simulink library "BAL_lib"  (Simulink 7.4)
settings: Solver=FixedStepDiscrete  StartTime=0.0  StopTime=Inf  FixedStep=0.01  RelTol=1e-3
undefined symbols (not defined in the file or in its folder): FCM_Charging_St, PACK_Const_CellNumOfPack, SCM_Charging_St
libraries: Defined_Functionality x3
settings Model: Creator=zhaoxiangri  LastModifiedBy=sunsijun

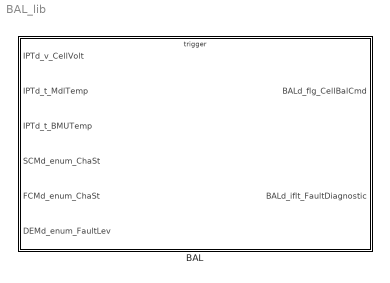
== system BAL_lib ==
  BAL : Subsystem  TreatAsAtomicUnit=on

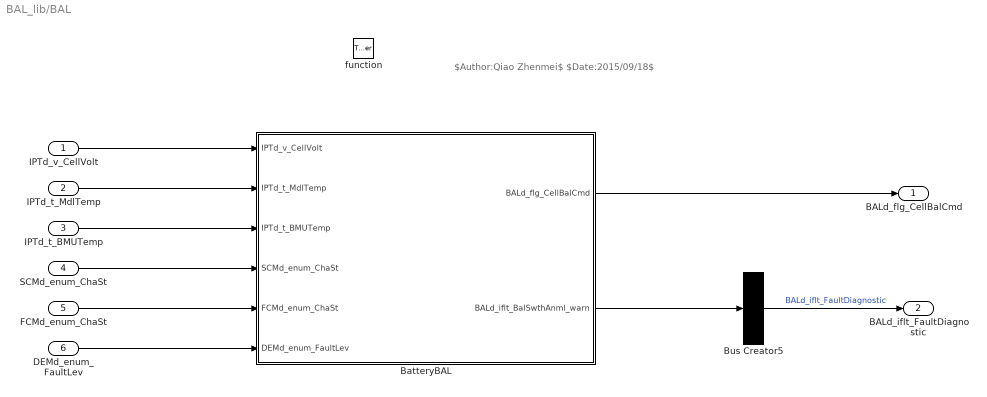
== system BAL_lib/BAL ==
  note: $Author:Qiao Zhenmei$
      | $Date:2015/09/18$
  IPTd_v_CellVolt : Inport  PortDimensions=[1 160]
  IPTd_t_MdlTemp : Inport  Port=2  DataType=single  OutDataTypeStr=single
  IPTd_t_BMUTemp : Inport  Port=3  DataType=single  OutDataTypeStr=single
  SCMd_enum_ChaSt : Inport  Port=4  DataType=uint8  OutDataTypeStr=uint8
  FCMd_enum_ChaSt : Inport  Port=5
  DEMd_enum_FaultLev : Inport  Port=6  DataType=uint8  OutDataTypeStr=uint8
  function : TriggerPort  TriggerType=function-call
  BatteryBAL : Subsystem  TreatAsAtomicUnit=on
  Bus Creator5 : BusCreator  Inputs=1
  BALd_flg_CellBalCmd : Outport
  BALd_iflt_FaultDiagnostic : Outport  Port=2  OutDataType=fixdt(1, 16)  OutScaling=2^0
  wires:
  Bus Creator5/1 -> BALd_iflt_FaultDiagnostic/1  "BALd_iflt_FaultDiagnostic"
  BatteryBAL/2(BALd_iflt_BalSwthAnml_warn) -> Bus Creator5/1
  IPTd_t_BMUTemp/1 -> BatteryBAL/3(IPTd_t_BMUTemp)
  BatteryBAL/1(BALd_flg_CellBalCmd) -> BALd_flg_CellBalCmd/1
  DEMd_enum_FaultLev/1 -> BatteryBAL/6(DEMd_enum_FaultLev)
  IPTd_t_MdlTemp/1 -> BatteryBAL/2(IPTd_t_MdlTemp)
  IPTd_v_CellVolt/1 -> BatteryBAL/1(IPTd_v_CellVolt)
  SCMd_enum_ChaSt/1 -> BatteryBAL/4(SCMd_enum_ChaSt)
  FCMd_enum_ChaSt/1 -> BatteryBAL/5(FCMd_enum_ChaSt)

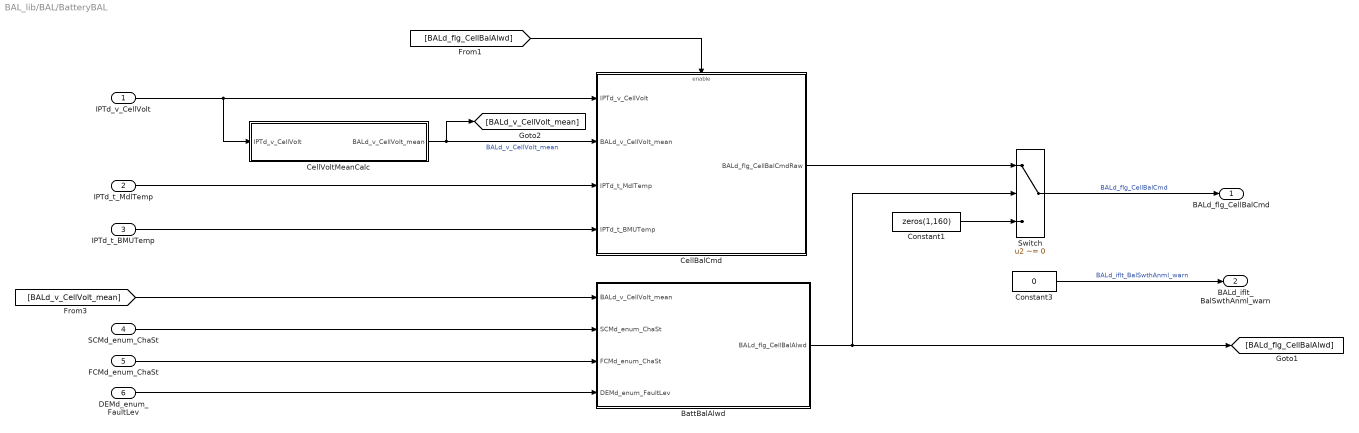
== system BAL_lib/BAL/BatteryBAL ==
  IPTd_v_CellVolt : Inport  DataType=single  OutDataTypeStr=single
  IPTd_t_MdlTemp : Inport  Port=2
  IPTd_t_BMUTemp : Inport  Port=3
  SCMd_enum_ChaSt : Inport  Port=4  DataType=uint8  OutDataTypeStr=uint8
  FCMd_enum_ChaSt : Inport  Port=5
  DEMd_enum_FaultLev : Inport  Port=6
  BattBalAlwd : Subsystem
  CellBalCmd : Subsystem
  CellVoltMeanCalc : Subsystem
  Constant1 : Constant  Value=zeros(1,160)  OutDataTypeMode=boolean  OutDataType=fixdt(1, 16)  OutScaling=2^0  OutDataTypeStr=boolean
  Constant3 : Constant  Value=0  OutDataTypeMode=boolean  OutDataTypeStr=boolean
  Switch : Switch  Criteria=u2 ~= 0  OutDataType=fixdt(1, 16)  OutScaling=2^0
  BALd_flg_CellBalCmd : Outport
  BALd_iflt_BalSwthAnml_warn : Outport  Port=2  OutDataType=fixdt(1, 16)  OutScaling=2^0  InitialOutput=0
  wires:
  [BALd_flg_CellBalAlwd] -> CellBalCmd/Enable
  CellBalCmd/1(BALd_flg_CellBalCmdRaw) -> Switch/1
  Constant1/1 -> Switch/3
  CellVoltMeanCalc/1(BALd_v_CellVolt_mean) -> [BALd_v_CellVolt_mean], CellBalCmd/2(BALd_v_CellVolt_mean)  "BALd_v_CellVolt_mean"
  Constant3/1 -> BALd_iflt_BalSwthAnml_warn/1  "BALd_iflt_BalSwthAnml_warn"
  IPTd_v_CellVolt/1 -> CellVoltMeanCalc/1(IPTd_v_CellVolt), CellBalCmd/1(IPTd_v_CellVolt)
  Switch/1 -> BALd_flg_CellBalCmd/1  "BALd_flg_CellBalCmd"
  IPTd_t_MdlTemp/1 -> CellBalCmd/3(IPTd_t_MdlTemp)
  IPTd_t_BMUTemp/1 -> CellBalCmd/4(IPTd_t_BMUTemp)
  BattBalAlwd/1(BALd_flg_CellBalAlwd) -> [BALd_flg_CellBalAlwd], Switch/2
  [BALd_v_CellVolt_mean] -> BattBalAlwd/1(BALd_v_CellVolt_mean)
  DEMd_enum_FaultLev/1 -> BattBalAlwd/4(DEMd_enum_FaultLev)
  SCMd_enum_ChaSt/1 -> BattBalAlwd/2(SCMd_enum_ChaSt)
  FCMd_enum_ChaSt/1 -> BattBalAlwd/3(FCMd_enum_ChaSt)

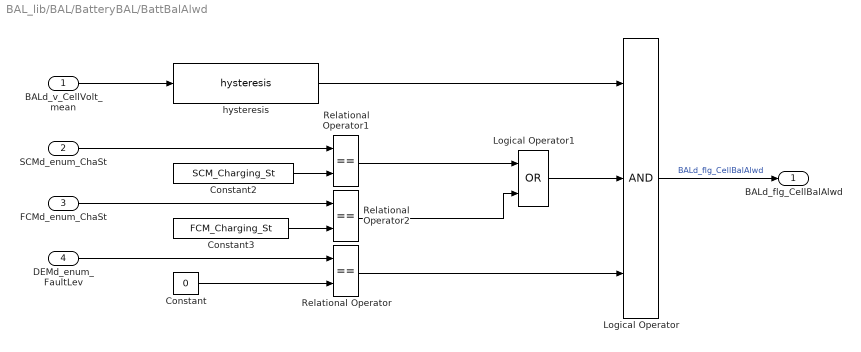
== system BAL_lib/BAL/BatteryBAL/BattBalAlwd ==
  BALd_v_CellVolt_mean : Inport
  SCMd_enum_ChaSt : Inport  Port=2  DataType=uint8  OutDataTypeStr=uint8
  FCMd_enum_ChaSt : Inport  Port=3
  DEMd_enum_FaultLev : Inport  Port=4
  Constant : Constant  Value=0  OutDataTypeMode=uint8  OutDataTypeStr=uint8
  Constant2 : Constant  Value=SCM_Charging_St  OutDataTypeMode=uint8  OutDataTypeStr=uint8
  Constant3 : Constant  Value=FCM_Charging_St  OutDataTypeMode=uint8  OutDataTypeStr=uint8
  Logical Operator : Logic  Inputs=3  AllPortsSameDT=off  OutDataTypeMode=boolean  OutDataTypeStr=boolean
  Logical Operator1 : Logic  Operator=OR  AllPortsSameDT=off  OutDataTypeMode=boolean  LogicDataType=fixdt(0, 8)  OutDataTypeStr=boolean
  Relational Operator : RelationalOperator  Operator===  LogicOutDataTypeMode=boolean  OutDataTypeStr=boolean
  Relational Operator1 : RelationalOperator  Operator===  LogicOutDataTypeMode=boolean  OutDataTypeStr=boolean
  Relational Operator2 : RelationalOperator  Operator===  LogicOutDataTypeMode=boolean  OutDataTypeStr=boolean
  hysteresis : Defined_Functionality/hysteresis  SystemSampleTime=-1  upper_limit=BALc_v_BalCellVoltOn  lower_limit=BALc_v_BalCellVoltOff
      settings: AttributesFormatString=[UPPER_LIMIT=%<upper_limit>]\n[LOWER_LIMIT=%<lower_limit>]
  BALd_flg_CellBalAlwd : Outport
  wires:
  hysteresis/1 -> Logical Operator/1
  Relational Operator2/1 -> Logical Operator1/2
  Logical Operator1/1 -> Logical Operator/2
  Constant3/1 -> Relational Operator2/2
  BALd_v_CellVolt_mean/1 -> hysteresis/1
  Logical Operator/1 -> BALd_flg_CellBalAlwd/1  "BALd_flg_CellBalAlwd"
  Relational Operator/1 -> Logical Operator/3
  Constant/1 -> Relational Operator/2
  DEMd_enum_FaultLev/1 -> Relational Operator/1
  FCMd_enum_ChaSt/1 -> Relational Operator2/1
  Relational Operator1/1 -> Logical Operator1/1
  Constant2/1 -> Relational Operator1/2
  SCMd_enum_ChaSt/1 -> Relational Operator1/1

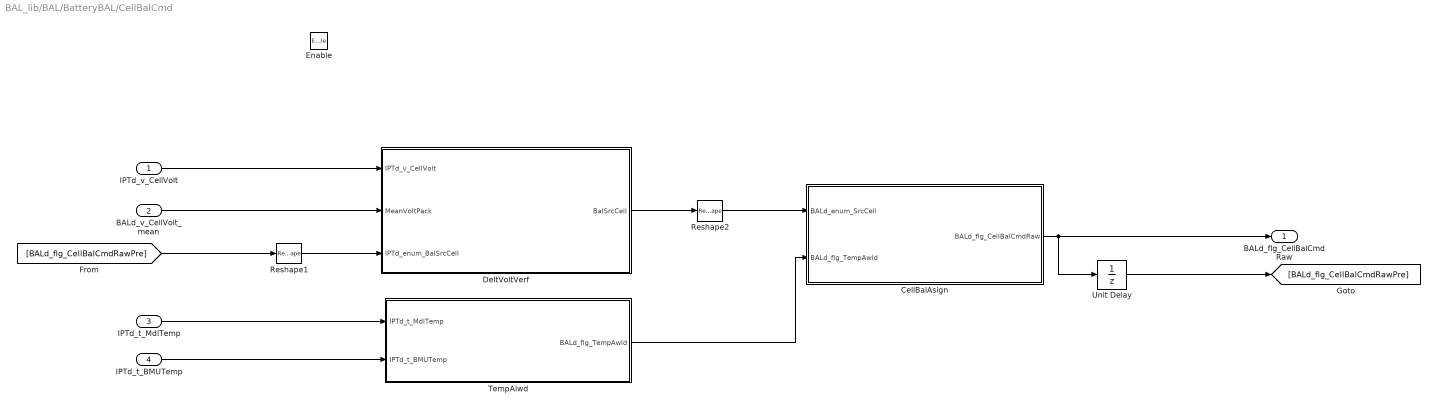
== system BAL_lib/BAL/BatteryBAL/CellBalCmd ==
  IPTd_v_CellVolt : Inport
  BALd_v_CellVolt_mean : Inport  Port=2
  IPTd_t_MdlTemp : Inport  Port=3
  IPTd_t_BMUTemp : Inport  Port=4
  Enable : EnablePort
  CellBalAsign : Subsystem
  DeltVoltVerf : Stateflow chart  TreatAsAtomicUnit=on
  Reshape1 : Reshape  OutputDimensionality=Customize  OutputDimensions=[5,32]
  Reshape2 : Reshape  OutputDimensionality=Row vector (2-D)  OutputDimensions=[40,4]
  TempAlwd : Subsystem
  Unit Delay : UnitDelay  SampleTime=-1
  BALd_flg_CellBalCmdRaw : Outport
  wires:
  [BALd_flg_CellBalCmdRawPre] -> Reshape1/1
  Unit Delay/1 -> [BALd_flg_CellBalCmdRawPre]
  Reshape2/1 -> CellBalAsign/1(BALd_enum_SrcCell)
  Reshape1/1 -> DeltVoltVerf/3(IPTd_enum_BalSrcCell)
  DeltVoltVerf/1(BalSrcCell) -> Reshape2/1
  TempAlwd/1(BALd_flg_TempAwld) -> CellBalAsign/2(BALd_flg_TempAwld)
  IPTd_t_MdlTemp/1 -> TempAlwd/1(IPTd_t_MdlTemp)
  IPTd_t_BMUTemp/1 -> TempAlwd/2(IPTd_t_BMUTemp)
  BALd_v_CellVolt_mean/1 -> DeltVoltVerf/2(MeanVoltPack)
  CellBalAsign/1(BALd_flg_CellBalCmdRaw) -> BALd_flg_CellBalCmdRaw/1, Unit Delay/1
  IPTd_v_CellVolt/1 -> DeltVoltVerf/1(IPTd_v_CellVolt)

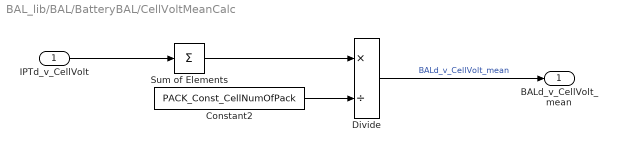
== system BAL_lib/BAL/BatteryBAL/CellVoltMeanCalc ==
  IPTd_v_CellVolt : Inport
  Constant2 : Constant  Value=PACK_Const_CellNumOfPack  OutDataTypeMode=uint8  OutDataTypeStr=uint8
  Divide : Product  Inputs=*/  OutDataType=fixdt(1, 16)  OutScaling=2^-10
  Sum of Elements : Sum  Inputs=+  OutDataType=fixdt(1, 16)  OutScaling=2^-10
  BALd_v_CellVolt_mean : Outport
  wires:
  Divide/1 -> BALd_v_CellVolt_mean/1  "BALd_v_CellVolt_mean"
  IPTd_v_CellVolt/1 -> Sum of Elements/1
  Constant2/1 -> Divide/2
  Sum of Elements/1 -> Divide/1

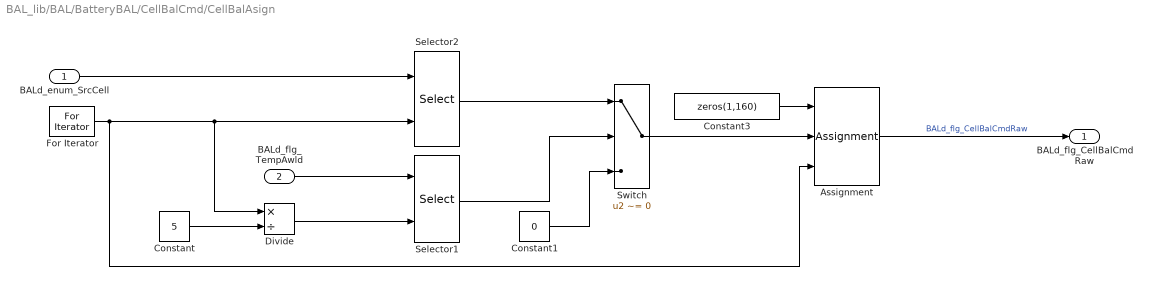
== system BAL_lib/BAL/BatteryBAL/CellBalCmd/CellBalAsign ==
  BALd_enum_SrcCell : Inport
  BALd_flg_TempAwld : Inport  Port=2
  Assignment : Assignment  IndexOptions=Index vector (port)  Indices=1  OutputSizes=1
  Constant : Constant  Value=5  OutDataTypeMode=uint8  OutDataType=fixdt(1, 16)  OutScaling=2^0  OutDataTypeStr=uint8
  Constant1 : Constant  Value=0  OutDataTypeMode=boolean  OutDataType=fixdt(1, 16)  OutScaling=2^0  OutDataTypeStr=boolean
  Constant3 : Constant  Value=zeros(1,160)  OutDataTypeMode=boolean  OutDataType=fixdt(1, 16)  OutScaling=2^0  OutDataTypeStr=boolean
  Divide : Product  Inputs=*/  OutDataTypeMode=uint8  OutDataType=fixdt(1, 16)  OutScaling=2^-10  OutDataTypeStr=uint8  RndMeth=Ceiling
  For Iterator : ForIterator  IterationLimit=160
  Selector1 : Selector  InputPortWidth=32  IndexOptions=Index vector (port)  Indices=[1 3]  OutputSizes=1
  Selector2 : Selector  InputPortWidth=160  IndexOptions=Index vector (port)  Indices=[1 3]  OutputSizes=1
  Switch : Switch  Criteria=u2 ~= 0  OutDataType=fixdt(1, 16)  OutScaling=2^0
  BALd_flg_CellBalCmdRaw : Outport
  wires:
  Switch/1 -> Assignment/2
  Constant1/1 -> Switch/3
  Selector2/1 -> Switch/1
  Selector1/1 -> Switch/2
  Divide/1 -> Selector1/2
  Constant/1 -> Divide/2
  BALd_enum_SrcCell/1 -> Selector2/1
  BALd_flg_TempAwld/1 -> Selector1/1
  For Iterator/1 -> Assignment/3, Divide/1, Selector2/2
  Assignment/1 -> BALd_flg_CellBalCmdRaw/1  "BALd_flg_CellBalCmdRaw"
  Constant3/1 -> Assignment/1

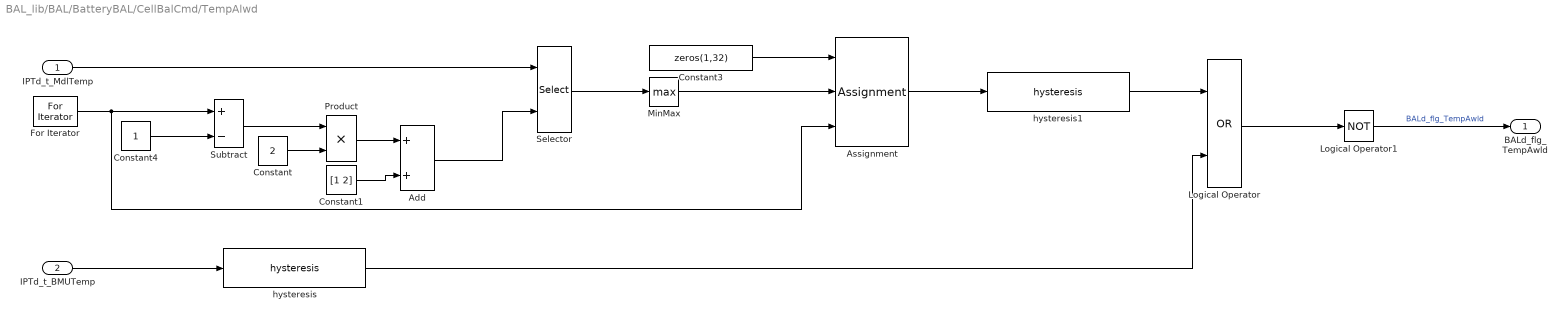
== system BAL_lib/BAL/BatteryBAL/CellBalCmd/TempAlwd ==
  IPTd_t_MdlTemp : Inport
  IPTd_t_BMUTemp : Inport  Port=2
  Add : Sum  OutDataType=fixdt(1, 16)  OutScaling=2^-10
  Assignment : Assignment  IndexOptions=Index vector (port)  Indices=1  OutputSizes=1
  Constant : Constant  Value=2  OutDataTypeMode=int32  OutDataType=fixdt(1, 16)  OutScaling=2^0  OutDataTypeStr=int32
  Constant1 : Constant  Value=[1 2]  OutDataTypeMode=uint8  OutDataType=fixdt(1, 16)  OutScaling=2^0  OutDataTypeStr=uint8
  Constant3 : Constant  Value=zeros(1,32)  OutDataType=fixdt(1, 16)  OutScaling=2^0  OutDataTypeStr=Inherit: Inherit via back propagation
  Constant4 : Constant  OutDataTypeMode=int32  OutDataType=fixdt(1, 16)  OutScaling=2^0  OutDataTypeStr=int32
  For Iterator : ForIterator  IterationLimit=32
  Logical Operator : Logic  Operator=OR  AllPortsSameDT=off  OutDataTypeMode=boolean  LogicDataType=fixdt(0, 8)  OutDataTypeStr=boolean
  Logical Operator1 : Logic  Operator=NOT  AllPortsSameDT=off  OutDataTypeMode=boolean  LogicDataType=fixdt(0, 8)  OutDataTypeStr=boolean
  MinMax : MinMax  Function=max  OutDataType=fixdt(1, 16)  OutScaling=2^0
  Product : Product  OutDataTypeMode=int32  OutDataType=fixdt(1, 16)  OutScaling=2^0  OutDataTypeStr=int32  RndMeth=Zero
  Selector : Selector  InputPortWidth=64  IndexOptions=Index vector (port)  Indices=[1 3]  OutputSizes=1
  Subtract : Sum  Inputs=+-  OutDataType=fixdt(1, 16)  OutScaling=2^-10
  hysteresis : Defined_Functionality/hysteresis  SystemSampleTime=-1  upper_limit=BALc_t_BalBMUTempOff  lower_limit=BALc_t_BalBMUTempOn
      settings: AttributesFormatString=[UPPER_LIMIT=%<upper_limit>]\n[LOWER_LIMIT=%<lower_limit>]
  hysteresis1 : Defined_Functionality/hysteresis  SystemSampleTime=-1  upper_limit=BALc_t_BalMdlTempOff  lower_limit=BALc_t_BalMdlTempOn
      settings: AttributesFormatString=[UPPER_LIMIT=%<upper_limit>]\n[LOWER_LIMIT=%<lower_limit>]
  BALd_flg_TempAwld : Outport
  wires:
  Logical Operator1/1 -> BALd_flg_TempAwld/1  "BALd_flg_TempAwld"
  hysteresis1/1 -> Logical Operator/1
  Constant4/1 -> Subtract/2
  Subtract/1 -> Product/1
  Logical Operator/1 -> Logical Operator1/1
  hysteresis/1 -> Logical Operator/2
  Constant3/1 -> Assignment/1
  Assignment/1 -> hysteresis1/1
  MinMax/1 -> Assignment/2
  Selector/1 -> MinMax/1
  Add/1 -> Selector/2
  Constant1/1 -> Add/2
  Product/1 -> Add/1
  Constant/1 -> Product/2
  For Iterator/1 -> Subtract/1, Assignment/3
  IPTd_t_MdlTemp/1 -> Selector/1
  IPTd_t_BMUTemp/1 -> hysteresis/1

== matlab function BAL/BatteryBAL/CellBalCmd/DeltVoltVerf ==
  data: IPTd_v_CellVolt input double size=[1 160]; MeanVoltPack input double; BalSrcCell output boolean size=[5 32]; IPTd_enum_BalSrcCell input double size=[5 32]; BALc_v_BalOffVoltDif_limit parameter double; BALc_v_BalOnVoltDif_limit parameter double; BALc_v_RepcBalOffVoltDif_limit parameter double; BALc_v_RepcBalOnVoltDif_limit parameter double
function BalSrcCell  = fcn(IPTd_v_CellVolt,MeanVoltPack, IPTd_enum_BalSrcCell,BALc_v_BalOffVoltDif_limit, BALc_v_BalOnVoltDif_limit, BALc_v_RepcBalOffVoltDif_limit, BALc_v_RepcBalOnVoltDif_limit)

%#initialization
BalSrcCell=IPTd_enum_BalSrcCell;
PrstBalSrcCell=IPTd_enum_BalSrcCell;
BALt_num_BalCellNum=sum(PrstBalSrcCell,1);
MinBalDeltVolt=[4 4 4 4];
BalBrekCell=0;


%calculate voltage difference
VoltDif=reshape(IPTd_v_CellVolt,5,32);
VoltDif=VoltDif-MeanVoltPack;

%%
[DeltVolt CellDim]=sort(VoltDif);
%To determine if the balancing cells should be closed.
for i=1:32;
    for j=5:-1:1;
        if PrstBalSrcCell(CellDim(j,i),i)==1;
          if VoltDif(CellDim(j,i),i)<=BALc_v_BalOffVoltDif_limit;
               BalSrcCell(CellDim(j,i),i)=0;
               BALt_num_BalCellNum(i)=BALt_num_BalCellNum(i)-1;
          else
              continue;
          end
        else
            continue;
        end
    end
end
%To determine if the unbalancing cells should be opened.
for k=1:32;
    for m=5:-1:1;
        if BALt_num_BalCellNum(1,k)<3;
            if PrstBalSrcCell(CellDim(m,k),k)==0;
               if VoltDif(CellDim(m,k),k)>=BALc_v_BalOnVoltDif_limit;
                  BalSrcCell(CellDim(m,k),k) =1;
                  BALt_num_BalCellNum(k)=BALt_num_BalCellNum(k)+1; 
               else
                   continue;                   
               end
            else
                continue;
            end
        else
            if PrstBalSrcCell(CellDim(m,k),k)==0;
                if VoltDif(CellDim(m,k),k)>=BALc_v_RepcBalOnVoltDif_limit;
%To caculate the balancing cells minimum voltage difference.
                    for jj=1:5;
                        if PrstBalSrcCell(jj,k)==1&&VoltDif(jj,k)<MinBalDeltVolt(1,k);
                           MinBalDeltVolt(1,k)=VoltDif(jj,k);
                           BalBrekCell=jj;
                        else
                        continue;
                        end
                    end
 %If the balancing cells minimum voltage difference<0.015V,replace it.
                    if MinBalDeltVolt(1,k)<BALc_v_RepcBalOffVoltDif_limit;
                   BalSrcCell(CellDim(m,k),k)=1;
                   BalSrcCell(BalBrekCell,k)=0;
                    else
                       break
                    end
                else
                    break
                end
            else
                continue
            end
        end
    end
end
